simulink model "samplesim"  (R2023a)
settings: Solver=VariableStepAuto  StartTime=0.0  StopTime=10.0  RelTol=1e-3
libraries: simulink_extras x4
settings Model: Creator=Sriram Sakthivel  LastModifiedBy=Sriram Sakthivel

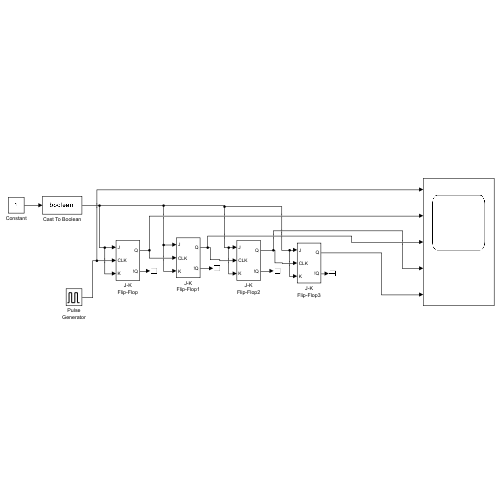
[thumbnail: Simulink's stored preview of the top-level diagram]
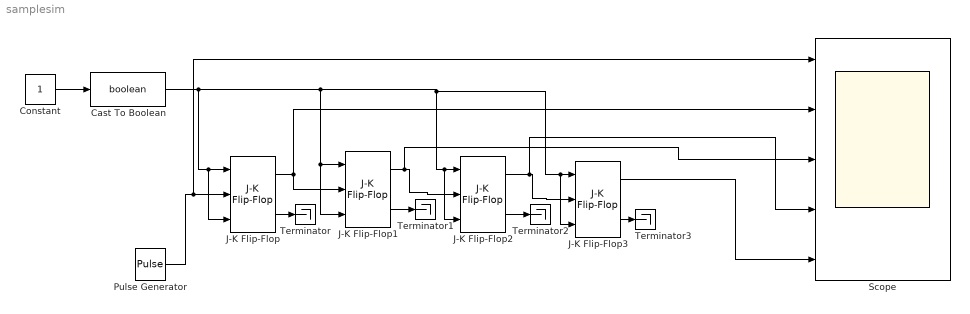
== system samplesim ==
  Cast To Boolean : DataTypeConversion  OutDataTypeStr=boolean  SaturateOnIntegerOverflow=off  RndMeth=Floor
  Constant : Constant
  J-K Flip-Flop{,1..3} (4 alike) : simulink_extras/Flip Flops/J-K Flip-Flop  initial_condition=0
  Pulse Generator : DiscretePulseGenerator  PulseType=Time based  Period=1  PulseWidth=5
  Scope : Scope  NumInputPorts=5
  Terminator{,1..3} (4 alike) : Terminator
  wires:
  J-K Flip-Flop/1 -> Scope/2, J-K Flip-Flop1/2
  Pulse Generator/1 -> Scope/1, J-K Flip-Flop/2
  J-K Flip-Flop/2 -> Terminator/1
  J-K Flip-Flop1/2 -> Terminator1/1
  J-K Flip-Flop2/2 -> Terminator2/1
  J-K Flip-Flop1/1 -> Scope/3, J-K Flip-Flop2/2
  J-K Flip-Flop3/2 -> Terminator3/1
  J-K Flip-Flop2/1 -> Scope/4, J-K Flip-Flop3/2
  Cast To Boolean/1 -> J-K Flip-Flop3/3, J-K Flip-Flop3/1, J-K Flip-Flop2/3, J-K Flip-Flop2/1, J-K Flip-Flop1/3, J-K Flip-Flop1/1, J-K Flip-Flop/3, J-K Flip-Flop/1
  Constant/1 -> Cast To Boolean/1
  J-K Flip-Flop3/1 -> Scope/5
